simulink model "RT_ueb3_2orig"  (R2013a)
settings: Solver=ode45  StartTime=0.0  StopTime=10.0  RelTol=1e-3
values from neighbouring files (symbols this model uses):
  k = 2    [rt_uebung2_post.m]
settings Model: Creator=mainster  LastModifiedBy=mainster

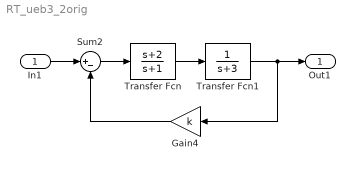
== system RT_ueb3_2orig ==
  In1 : Inport
  Gain4 : Gain  Gain=k
  Sum2 : Sum  Inputs=|+-
  Transfer Fcn : TransferFcn  Numerator=[1 2]  Denominator=[1 1]
  Transfer Fcn1 : TransferFcn  Denominator=[1 3]
  Out1 : Outport
  wires:
  Sum2/1 -> Transfer Fcn/1
  Gain4/1 -> Sum2/2
  In1/1 -> Sum2/1
  Transfer Fcn/1 -> Transfer Fcn1/1
  Transfer Fcn1/1 -> Gain4/1, Out1/1
